simulink model "LoadFlow_and_Fault_Analysis_of_7Bus_System__25032026"  (R2024b)
settings: Solver=VariableStepAuto  StartTime=0.0  StopTime=10.0  RelTol=1e-3
InitFcn:
  | R12 = 0.5025
  | R23 = 0.4020
  | R34 = 0.3660
  | R25 = 0.3840
  | R56 = 0.8910
  | R27 = 0.2872
  | R17 = 0.5025
  | R46 = 0.5025
  | 
  | X12 = 0.3025
  | X23 = 0.2510
  | X34 = 0.1864
  | X25 = 0.1965
  | X56 = 0.7050
  | X27 = 0.4088
  | X17 = 0.3025
  | X46 = 0.3025
  | 
  | P12 = 1e6
  | P23 = 0.9e6
  | P34 = 2.5e6
  | P25 = 1.2e6
  | P56 = 1.05e6
  | P27 = 2e6
  | P17 = 0
  | P46 = 0
  | 
  | Q12 = 0.6e6
  | Q23 = 0.5e6
  | Q34 = 1.2e6
  | Q25 = 0.95e6
  | Q56 = 0.78e6
  | Q27 = 1.15e6
  | Q17 = 0
  | Q46 = 0
undefined symbols (not defined in the file or in its folder): C23, C67
libraries: spsThreePhaseSeriesRLCBranchLib x8, spsLoadFlowBusLib x7, spsThreePhaseVIMeasurementLib x7, spsThreePhaseSeriesRLCLoadLib x6, spsRMSLib x4, spsThreePhaseBreakerLib x2, spsThreePhaseFaultLib x1, spsThreePhaseSourceLib x1, sps_lib x1
settings Model: Creator=cachu  LastModifiedBy=cachu

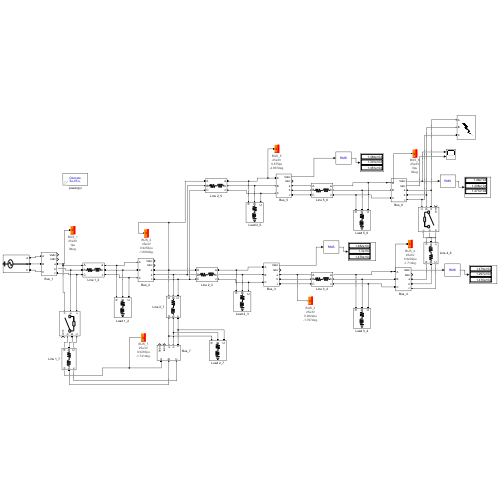
[thumbnail: Simulink's stored preview of the top-level diagram]
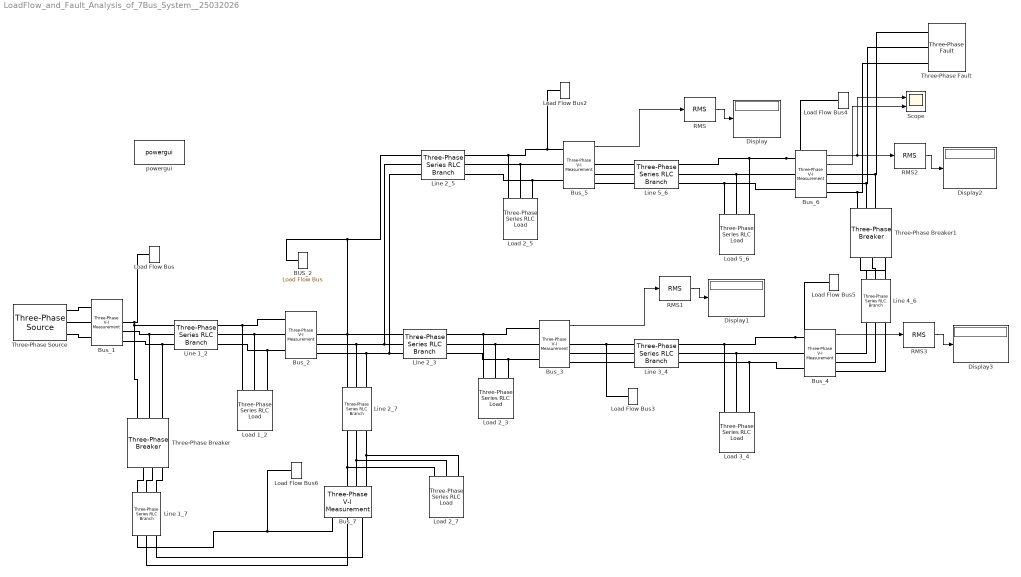
== system LoadFlow_and_Fault_Analysis_of_7Bus_System__25032026 ==
  " Load 2_5" : spsThreePhaseSeriesRLCLoadLib/Three-Phase Series RLC Load  LConnTagsString=A|B|C  Configuration=Y (grounded)  NominalVoltage=(25000)*0.874997  Vabc=[1e3 1e3 1e3]  Vabcp=[1e3 1e3 1e3]  NominalFrequency=50  UnbalancedPower=off  ActivePower=1200000  InductivePower=950000  CapacitivePower=0  Pabc=[10e3 9e3 11e3]  QLabc=[100 90 110]  QCabc=[100 90 110]  Pabcp=[10e3 9e3 11e3]  QLabcp=[100 90 110]  QCabcp=[100 90 110]  Measurements=None  LoadType=constant PQ
  BUS_2 : spsLoadFlowBusLib/Load Flow Bus  LConnTagsString=a  Phases=single  Connectors=on one side  ID=BUS_2  Vbase=25e3  Vref=1  Vangle=0  VLF=0.9253  VLFb=1  VLFc=1  angleLF=-1.689  angleLFb=0  angleLFc=0
  Bus_{1..6} (6 alike) : spsThreePhaseVIMeasurementLib/Three-Phase V-I Measurement  VoltageMeasurement=phase-to-ground  SetLabelV=off  LabelV=Vabc  Vpu=off  VpuLL=off  CurrentMeasurement=yes  SetLabelI=off  LabelI=Iabc  Ipu=off  Pbase=100e6  Vbase=500e3  OutputType=Complex  PhasorSimulation=off  PSBequivalent=0
  "Bus_7 " : spsThreePhaseVIMeasurementLib/Three-Phase V-I Measurement  VoltageMeasurement=phase-to-ground  SetLabelV=off  LabelV=Vabc  Vpu=off  VpuLL=off  CurrentMeasurement=yes  SetLabelI=off  LabelI=Iabc  Ipu=off  Pbase=100e6  Vbase=500e3  OutputType=Complex  PhasorSimulation=off  PSBequivalent=0
  Display{,1..3} (4 alike) : Display
  Line 1_2 : spsThreePhaseSeriesRLCBranchLib/Three-Phase Series RLC Branch  LConnTagsString=A|B|C  RConnTagsString=A|B|C  BranchType=RL  Resistance=R12  Inductance=X12/314  Capacitance=0  Measurements=None
  Line 1_7 : spsThreePhaseSeriesRLCBranchLib/Three-Phase Series RLC Branch  LConnTagsString=A|B|C  RConnTagsString=A|B|C  BranchType=RL  Resistance=R17  Inductance=X17/314  Capacitance=1e-6  Measurements=None
  Line 2_3 : spsThreePhaseSeriesRLCBranchLib/Three-Phase Series RLC Branch  LConnTagsString=A|B|C  RConnTagsString=A|B|C  BranchType=RL  Resistance=R23  Inductance=X23/314  Capacitance=C23  Measurements=None
  Line 2_5 : spsThreePhaseSeriesRLCBranchLib/Three-Phase Series RLC Branch  LConnTagsString=A|B|C  RConnTagsString=A|B|C  BranchType=RL  Resistance=R25  Inductance=X25/314  Capacitance=1e-6  Measurements=None
  Line 2_7 : spsThreePhaseSeriesRLCBranchLib/Three-Phase Series RLC Branch  LConnTagsString=A|B|C  RConnTagsString=A|B|C  BranchType=RL  Resistance=R27  Inductance=X27/314  Capacitance=C67  Measurements=None
  Line 3_4 : spsThreePhaseSeriesRLCBranchLib/Three-Phase Series RLC Branch  LConnTagsString=A|B|C  RConnTagsString=A|B|C  BranchType=RL  Resistance=R34  Inductance=X34/314  Capacitance=1e-6  Measurements=None
  Line 4_6 : spsThreePhaseSeriesRLCBranchLib/Three-Phase Series RLC Branch  LConnTagsString=A|B|C  RConnTagsString=A|B|C  BranchType=RL  Resistance=R46  Inductance=X46/314  Capacitance=1e-6  Measurements=None
  Line 5_6 : spsThreePhaseSeriesRLCBranchLib/Three-Phase Series RLC Branch  LConnTagsString=A|B|C  RConnTagsString=A|B|C  BranchType=RL  Resistance=R56  Inductance=X56/314  Capacitance=1e-6  Measurements=None
  Load 1_2 : spsThreePhaseSeriesRLCLoadLib/Three-Phase Series RLC Load  LConnTagsString=A|B|C  Configuration=Y (grounded)  NominalVoltage=(25000)*0.925331  Vabc=[1e3 1e3 1e3]  Vabcp=[1e3 1e3 1e3]  NominalFrequency=50  UnbalancedPower=off  ActivePower=1000000  InductivePower=600000  CapacitivePower=0  Pabc=[10e3 9e3 11e3]  QLabc=[100 90 110]  QCabc=[100 90 110]  Pabcp=[10e3 9e3 11e3]  QLabcp=[100 90 110]  QCabcp=[100 90 110]  Measurements=None  LoadType=constant PQ
  Load 2_3 : spsThreePhaseSeriesRLCLoadLib/Three-Phase Series RLC Load  LConnTagsString=A|B|C  Configuration=Y (grounded)  NominalVoltage=(25000)*0.922214  Vabc=[1e3 1e3 1e3]  Vabcp=[1e3 1e3 1e3]  NominalFrequency=50  UnbalancedPower=off  ActivePower=900000  InductivePower=500000  CapacitivePower=0  Pabc=[10e3 9e3 11e3]  QLabc=[100 90 110]  QCabc=[100 90 110]  Pabcp=[10e3 9e3 11e3]  QLabcp=[100 90 110]  QCabcp=[100 90 110]  Measurements=None  LoadType=constant PQ
  Load 2_7 : spsThreePhaseSeriesRLCLoadLib/Three-Phase Series RLC Load  LConnTagsString=A|B|C  Configuration=Y (grounded)  NominalVoltage=(25000)*0.92352  Vabc=[1e3 1e3 1e3]  Vabcp=[1e3 1e3 1e3]  NominalFrequency=50  UnbalancedPower=off  ActivePower=2000000  InductivePower=1150000  CapacitivePower=0  Pabc=[10e3 9e3 11e3]  QLabc=[100 90 110]  QCabc=[100 90 110]  Pabcp=[10e3 9e3 11e3]  QLabcp=[100 90 110]  QCabcp=[100 90 110]  Measurements=None  LoadType=constant PQ
  Load 3_4 : spsThreePhaseSeriesRLCLoadLib/Three-Phase Series RLC Load  LConnTagsString=A|B|C  Configuration=Y (grounded)  NominalVoltage=(25000)*0.920235  Vabc=[1e3 1e3 1e3]  Vabcp=[1e3 1e3 1e3]  NominalFrequency=50  UnbalancedPower=off  ActivePower=2500000  InductivePower=1200000  CapacitivePower=0  Pabc=[10e3 9e3 11e3]  QLabc=[100 90 110]  QCabc=[100 90 110]  Pabcp=[10e3 9e3 11e3]  QLabcp=[100 90 110]  QCabcp=[100 90 110]  Measurements=None  LoadType=constant PQ
  Load 5_6 : spsThreePhaseSeriesRLCLoadLib/Three-Phase Series RLC Load  LConnTagsString=A|B|C  Configuration=Y (grounded)  NominalVoltage=25e3  Vabc=[1e3 1e3 1e3]  Vabcp=[1e3 1e3 1e3]  NominalFrequency=50  UnbalancedPower=off  ActivePower=1050000  InductivePower=780000  CapacitivePower=0  Pabc=[10e3 9e3 11e3]  QLabc=[100 90 110]  QCabc=[100 90 110]  Pabcp=[10e3 9e3 11e3]  QLabcp=[100 90 110]  QCabcp=[100 90 110]  Measurements=None  LoadType=constant PQ
  Load Flow Bus : spsLoadFlowBusLib/Load Flow Bus  LConnTagsString=a  Phases=single  Connectors=on one side  ID=BUS_1  Vbase=25e3  Vref=1  Vangle=0  VLF=1  VLFb=1  VLFc=1  angleLF=0  angleLFb=0  angleLFc=0
  Load Flow Bus2 : spsLoadFlowBusLib/Load Flow Bus  LConnTagsString=a  Phases=single  Connectors=on one side  ID=BUS_5  Vbase=25e3  Vref=1  Vangle=0  VLF=0.875  VLFb=1  VLFc=1  angleLF=-2.867  angleLFb=0  angleLFc=0
  Load Flow Bus3 : spsLoadFlowBusLib/Load Flow Bus  LConnTagsString=a  Phases=single  Connectors=on one side  ID=BUS_3  Vbase=25e3  Vref=1  Vangle=0  VLF=0.9222  VLFb=1  VLFc=1  angleLF=-1.707  angleLFb=0  angleLFc=0
  Load Flow Bus4 : spsLoadFlowBusLib/Load Flow Bus  LConnTagsString=a  Phases=single  Connectors=on one side  ID=BUS_6  Vbase=25e3  Vref=1  Vangle=0  VLF=0  VLFb=1  VLFc=1  angleLF=0  angleLFb=0  angleLFc=0
  Load Flow Bus5 : spsLoadFlowBusLib/Load Flow Bus  LConnTagsString=a  Phases=single  Connectors=on one side  ID=BUS_4  Vbase=25e3  Vref=1  Vangle=0  VLF=0.9202  VLFb=1  VLFc=1  angleLF=-1.71  angleLFb=0  angleLFc=0
  Load Flow Bus6 : spsLoadFlowBusLib/Load Flow Bus  LConnTagsString=a  Phases=single  Connectors=on one side  ID=BUS_7  Vbase=25e3  Vref=1  Vangle=0  VLF=0.9235  VLFb=1  VLFc=1  angleLF=-1.741  angleLFb=0  angleLFc=0
  RMS{,1..3} (4 alike) : spsRMSLib/RMS  TrueRMS=on  Freq=60  RMSInit=120  Ts=0
  Scope : Scope  NumInputPorts=2
  Three-Phase Breaker : spsThreePhaseBreakerLib/Three-Phase Breaker  InitialState=open  SwitchA=on  SwitchB=on  SwitchC=on  SwitchTimes="[1/60  5/60]"  External=on  BreakerResistance=0.01  SnubberResistance=1e6  SnubberCapacitance=inf  Measurements=None
  Three-Phase Breaker1 : spsThreePhaseBreakerLib/Three-Phase Breaker  InitialState=open  SwitchA=on  SwitchB=on  SwitchC=on  SwitchTimes="[1/60  5/60]"  External=on  BreakerResistance=0.01  SnubberResistance=1e6  SnubberCapacitance=inf  Measurements=None
  Three-Phase Fault : spsThreePhaseFaultLib/Three-Phase Fault  InitialStates=0  FaultA=on  FaultB=off  FaultC=off  GroundFault=on  SwitchTimes=[0.5 0.6]  External=off  SwitchStatus=NaN  FaultResistance=0.001  GroundResistance=10  SnubberResistance=1e6  SnubberCapacitance=inf  Measurements=None
  Three-Phase Source : spsThreePhaseSourceLib/Three-Phase Source  InternalConnection=Yg  VoltagePhases=off  Voltage=(25000)*1  PhaseAngle=0  Voltage_phases=[25e3 25e3 25e3]/sqrt(3)  PhaseAngles_phases=[0 -120 +120]  Frequency=50  NonIdealSource=off  SpecifyImpedance=off  Resistance=0.8929  Inductance=16.58e-3  ShortCircuitLevel=100e6  BaseVoltage=25e3  XRratio=7  BusType=swing  Pref=10000  Qref=0  Prefabc=[10e3, 10e3, 10e3]  Qrefabc=[0, 0, 0]  Qmin=-Inf  Qmax=Inf
  powergui : sps_lib/powergui  Priority=1  SimulationMode=Discrete  SampleTime=50e-6  frequency=60  Iterations=50  frequencyindice=50  Pbase=100e6  ErrMax=1e-4  UnitsV=kV  UnitsW=MW  buscounter=0  FunctionMessages=off  echomessages=off  EnableUseOfTLC=off  CurrentSourceSwitches=off  DisableSnubberDevices=off  DisableRonSwitches=off  DisableVfSwitches=off  DisplayEquations=off  AutomaticDiscreteSolvers=off  SolverType=Tustin/Backward Euler (TBE)  Interpol=off  ExternalGateDelay=off  methode=off  Ts=100  x0status=blocks  SPID=on  SwTol=0  HookPort=off  NonlinearTolerance=1e-4  nMaxIteration=100  ContinueOnMaxIteration=off  RestoreLinks=warning  ResistiveCurrentMeasurement=off  Frange=[0:2:500]  Ylog=off  Xlog=on  ShowGrid=off  save=off  variable=ZData  structure=0  ZoomFFT=off  StartTime=0.0  cycles=1  DisplayStyle=1  fundamental=60  FreqAxis=off  MaxFrequency=1000  frequencyindicesteady=1  RmsSteady=1  display=off
  wires:
  RMS/1 -> Display/1
  Bus_5/1 -> RMS/1
  Bus_3/1 -> RMS1/1
  RMS1/1 -> Display1/1
  Bus_6/1 -> Scope/1, RMS2/1
  RMS2/1 -> Display2/1
  Bus_4/1 -> RMS3/1
  RMS3/1 -> Display3/1
  Bus_6/2 -> Scope/2
  connections:
  Bus_1/LConn1 -- Three-Phase Source/RConn1
  Bus_1/LConn2 -- Three-Phase Source/RConn2
  Bus_1/LConn3 -- Three-Phase Source/RConn3
  Line 1_2/LConn1 -- Load Flow Bus/LConn1 -- Bus_1/RConn1 -- Three-Phase Breaker/RConn1
  Line 1_2/LConn2 -- Bus_1/RConn2 -- Three-Phase Breaker/RConn2
  Line 1_2/LConn3 -- Bus_1/RConn3 -- Three-Phase Breaker/RConn3
  Bus_2/LConn3 -- Line 1_2/RConn3 -- Load 1_2/LConn3
  Bus_2/LConn2 -- Line 1_2/RConn2 -- Load 1_2/LConn2
  Bus_2/LConn1 -- Line 1_2/RConn1 -- Load 1_2/LConn1
  "Bus_7 "/RConn3 -- Line 2_7/RConn3 -- Load 2_7/LConn3
  "Bus_7 "/RConn2 -- Line 2_7/RConn2 -- Load 2_7/LConn2
  "Bus_7 "/RConn1 -- Line 2_7/RConn1 -- Load 2_7/LConn1
  "Bus_7 "/LConn1 -- Line 1_7/RConn1 -- Load Flow Bus6/LConn1
  Line 2_3/LConn1 -- Line 2_5/LConn1 -- BUS_2/LConn1 -- Line 2_7/LConn1 -- Bus_2/RConn1
  Line 2_3/LConn2 -- Line 2_7/LConn2 -- Bus_2/RConn2 -- Line 2_5/LConn2
  Line 2_3/LConn3 -- Line 2_7/LConn3 -- Bus_2/RConn3 -- Line 2_5/LConn3
  Bus_5/LConn2 -- Line 2_5/RConn2 -- " Load 2_5"/LConn2
  Line 2_5/RConn1 -- " Load 2_5"/LConn1 -- Load Flow Bus2/LConn1 -- Bus_5/LConn1
  Line 2_5/RConn3 -- Bus_5/LConn3 -- " Load 2_5"/LConn3
  Bus_3/LConn2 -- Line 2_3/RConn2 -- Load 2_3/LConn2
  Bus_3/LConn1 -- Line 2_3/RConn1 -- Load 2_3/LConn1
  Load 2_3/LConn3 -- Line 2_3/RConn3 -- Bus_3/LConn3
  Load Flow Bus3/LConn1 -- Bus_3/RConn1 -- Line 3_4/LConn1
  Line 5_6/LConn1 -- Bus_5/RConn1
  Line 5_6/LConn2 -- Bus_5/RConn2
  Line 5_6/LConn3 -- Bus_5/RConn3
  Line 3_4/LConn2 -- Bus_3/RConn2
  Line 3_4/LConn3 -- Bus_3/RConn3
  Bus_4/LConn2 -- Load 3_4/LConn2 -- Line 3_4/RConn2
  Line 3_4/RConn3 -- Bus_4/LConn3 -- Load 3_4/LConn3
  Bus_4/LConn1 -- Load 3_4/LConn1 -- Line 3_4/RConn1 -- Load Flow Bus5/LConn1
  Line 4_6/LConn1 -- Bus_4/RConn1
  Line 4_6/LConn2 -- Bus_4/RConn2
  Line 4_6/LConn3 -- Bus_4/RConn3
  Bus_6/LConn2 -- Line 5_6/RConn2 -- Load 5_6/LConn2
  Bus_6/LConn1 -- Load Flow Bus4/LConn1 -- Line 5_6/RConn1 -- Load 5_6/LConn3
  Line 5_6/RConn3 -- Load 5_6/LConn1 -- Bus_6/LConn3
  Bus_6/RConn1 -- Three-Phase Fault/LConn1 -- Three-Phase Breaker1/LConn1
  Bus_6/RConn2 -- Three-Phase Fault/LConn2 -- Three-Phase Breaker1/LConn2
  Bus_6/RConn3 -- Three-Phase Fault/LConn3 -- Three-Phase Breaker1/LConn3
  Three-Phase Breaker1/RConn1 -- Line 4_6/RConn1
  Three-Phase Breaker1/RConn3 -- Line 4_6/RConn3
  Three-Phase Breaker1/RConn2 -- Line 4_6/RConn2
  Line 1_7/LConn2 -- Three-Phase Breaker/LConn2
  Three-Phase Breaker/LConn3 -- Line 1_7/LConn3
  Line 1_7/LConn1 -- Three-Phase Breaker/LConn1
  "Bus_7 "/LConn2 -- Line 1_7/RConn2
  Line 1_7/RConn3 -- "Bus_7 "/LConn3
